simulink model "Solar_Voltage_Project"  (R2024a)
settings: Solver=VariableStepAuto  StartTime=0.0  StopTime=86400  RelTol=1e-3
libraries: spsControlledCurrentSourceLib x1, spsGroundLib x1, spsSeriesRLCBranchLib x1, spsThreePhaseParallelRLCBranchLib x1, spsThreePhaseSeriesRLCLoadLib x1, spsThreePhaseSourceLib x1, spsVoltageMeasurementLib x1, sps_lib x1
settings Model: Creator=CHANUPA  LastModifiedBy=CHANUPA

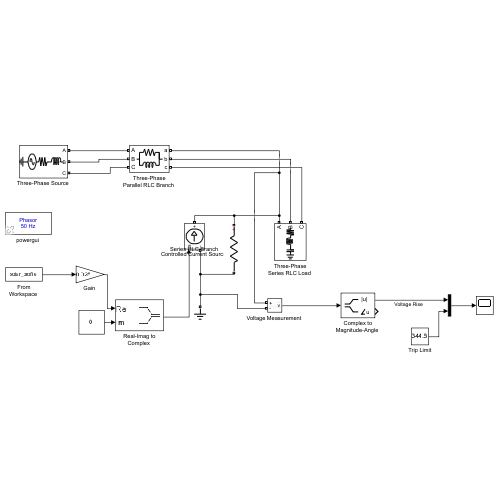
[thumbnail: Simulink's stored preview of the top-level diagram]
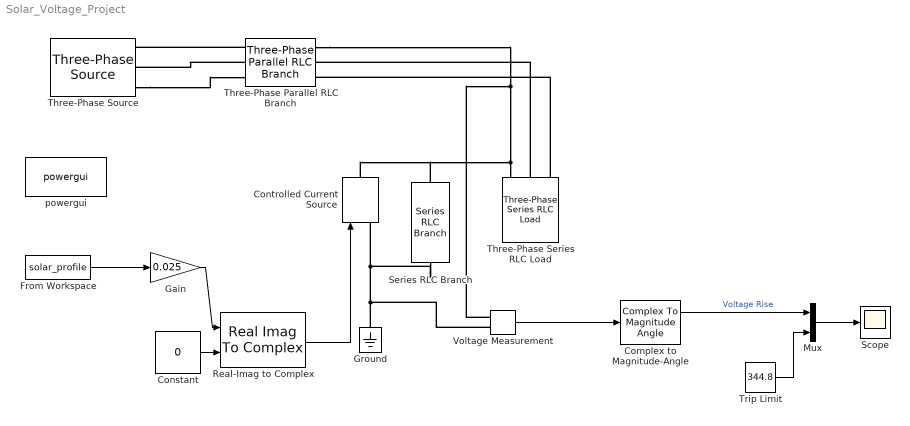
== system Solar_Voltage_Project ==
  "Complex to Magnitude-Angle " : ComplexToMagnitudeAngle
  Constant : Constant  Value=0
  "Controlled Current Source " : spsControlledCurrentSourceLib/Controlled Current Source  Initialize=on  Source_Type=AC  Amplitude=0  Phase=0  Frequency=0  Measurements=None
  "From Workspace " : FromWorkspace  VariableName=solar_profile  OutputAfterFinalValue=Setting to zero
  "Gain " : Gain  Gain=0.025
  Ground : spsGroundLib/Ground  LConnTagsString=a
  Mux : Mux  Inputs=2
  "Real-Imag to Complex " : RealImagToComplex
  Scope : Scope
  "Series RLC Branch " : spsSeriesRLCBranchLib/Series RLC Branch  LConnTagsString=__new0  RConnTagsString=__new0  BranchType=R  Resistance=100000  Inductance=1e-3  SetiL0=off  InitialCurrent=0  Capacitance=1e-6  Setx0=off  InitialVoltage=0  Measurements=None
  "Three-Phase Parallel RLC Branch " : spsThreePhaseParallelRLCBranchLib/Three-Phase Parallel RLC Branch  LConnTagsString=A|B|C  RConnTagsString=A|B|C  BranchType=RL  Resistance=0.22  Inductance=0.125e-3  Capacitance=inf  Measurements=None
  "Three-Phase Series RLC Load " : spsThreePhaseSeriesRLCLoadLib/Three-Phase Series RLC Load  LConnTagsString=A|B|C  Configuration=Y (grounded)  NominalVoltage=400  Vabc=[1e3 1e3 1e3]  Vabcp=[1e3 1e3 1e3]  NominalFrequency=50  UnbalancedPower=off  ActivePower=2000  InductivePower=100  CapacitivePower=100  Pabc=[10e3 9e3 11e3]  QLabc=[100 90 110]  QCabc=[100 90 110]  Pabcp=[10e3 9e3 11e3]  QLabcp=[100 90 110]  QCabcp=[100 90 110]  Measurements=None  LoadType=constant Z
  "Three-Phase Source " : spsThreePhaseSourceLib/Three-Phase Source  InternalConnection=Yg  VoltagePhases=off  Voltage=400  PhaseAngle=0  Voltage_phases=[25e3 25e3 25e3]/sqrt(3)  PhaseAngles_phases=[0 -120 +120]  Frequency=50  NonIdealSource=on  SpecifyImpedance=off  Resistance=0.8929  Inductance=16.58e-3  ShortCircuitLevel=100e6  BaseVoltage=25e3  XRratio=7  BusType=swing  Pref=10e3  Qref=0  Prefabc=[10e3, 10e3, 10e3]  Qrefabc=[0, 0, 0]  Qmin=-inf  Qmax=inf
  Trip Limit : Constant  Value=344.8
  "Voltage Measurement " : spsVoltageMeasurementLib/Voltage Measurement  PhasorSimulation=on  OutputType=Complex  PSBequivalent=0
  "powergui " : sps_lib/powergui  Priority=1  SimulationMode=Phasor  SampleTime=50e-6  frequency=50  Iterations=50  frequencyindice=50  Pbase=100e6  ErrMax=1e-4  UnitsV=kV  UnitsW=MW  buscounter=0  FunctionMessages=off  echomessages=off  EnableUseOfTLC=off  CurrentSourceSwitches=off  DisableSnubberDevices=off  DisableRonSwitches=off  DisableVfSwitches=off  DisplayEquations=off  AutomaticDiscreteSolvers=off  SolverType=Tustin/Backward Euler (TBE)  Interpol=off  ExternalGateDelay=off  methode=off  Ts=100  x0status=blocks  SPID=on  SwTol=0  HookPort=off  NonlinearTolerance=1e-4  nMaxIteration=100  ContinueOnMaxIteration=off  RestoreLinks=warning  ResistiveCurrentMeasurement=off  Frange=[0:2:500]  Ylog=off  Xlog=on  ShowGrid=off  save=off  variable=ZData  structure=0  ZoomFFT=off  StartTime=0.0  cycles=1  DisplayStyle=1  fundamental=60  FreqAxis=off  MaxFrequency=1000  frequencyindicesteady=1  RmsSteady=1  display=off
  wires:
  "From Workspace "/1 -> "Gain "/1
  "Voltage Measurement "/1 -> "Complex to Magnitude-Angle "/1
  "Gain "/1 -> "Real-Imag to Complex "/1
  Constant/1 -> "Real-Imag to Complex "/2
  "Real-Imag to Complex "/1 -> "Controlled Current Source "/1
  Trip Limit/1 -> Mux/2
  "Complex to Magnitude-Angle "/1 -> Mux/1  "Voltage Rise"
  Mux/1 -> Scope/1
  connections:
  "Three-Phase Parallel RLC Branch "/LConn1 -- "Three-Phase Source "/RConn1
  "Three-Phase Parallel RLC Branch "/LConn2 -- "Three-Phase Source "/RConn2
  "Three-Phase Source "/RConn3 -- "Three-Phase Parallel RLC Branch "/LConn3
  Ground/LConn1 -- "Voltage Measurement "/LConn2 -- "Series RLC Branch "/RConn1 -- "Controlled Current Source "/LConn1
  "Three-Phase Series RLC Load "/LConn2 -- "Three-Phase Parallel RLC Branch "/RConn2
  "Three-Phase Series RLC Load "/LConn3 -- "Three-Phase Parallel RLC Branch "/RConn3
  "Three-Phase Parallel RLC Branch "/RConn1 -- "Voltage Measurement "/LConn1 -- "Controlled Current Source "/RConn1 -- "Series RLC Branch "/LConn1 -- "Three-Phase Series RLC Load "/LConn1
